simulink model "myexp5_3"  (R2022a)
settings: Solver=VariableStepAuto  StartTime=0.0  StopTime=100000  RelTol=1e-3
values from neighbouring files (symbols this model uses):
  M = n_list(i)    [exp5h.m]
libraries: commblkcod2 x2, commrandsrc3 x1, commchan3 x1, commsink2 x1
settings Model: Creator=惠普  LastModifiedBy=惠普

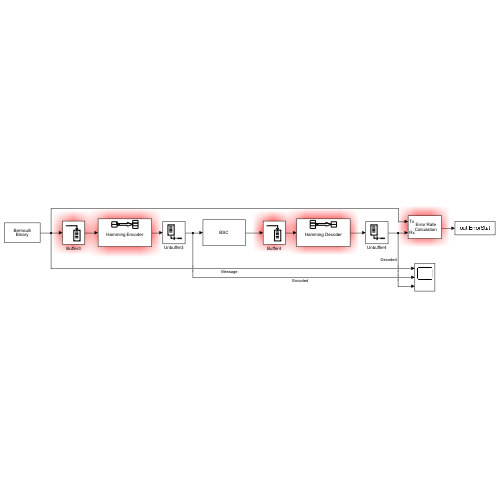
[thumbnail: Simulink's stored preview of the top-level diagram]
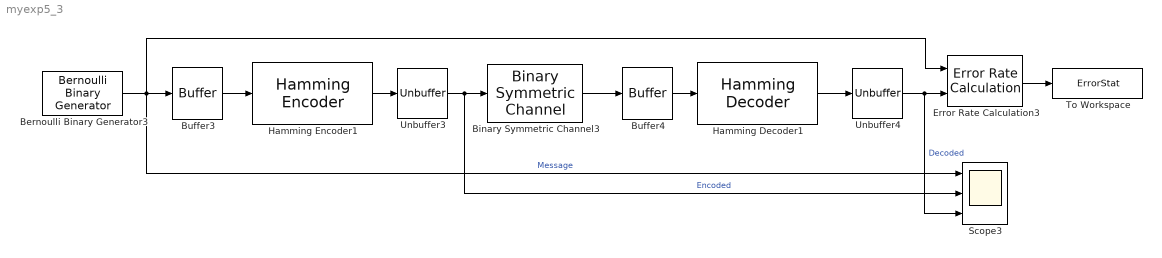
== system myexp5_3 ==
  Bernoulli Binary Generator3 : commrandsrc3/Bernoulli Binary Generator  ProbabilityOfZero=0.5  SeedSource=Auto  Seed=0  SampleTime=1  SamplesPerFrame=1  OutputDataType=double  SimulateUsing=Interpreted execution
  Binary Symmetric Channel3 : commchan3/Binary Symmetric Channel  ErrorProbability=eprob  ErrorVectorOutputPort=off  OutputDataType=double  OutputDataTypeSL=double  Seed=137  SimulateUsing=Code generation
      settings: SourceProductBaseCode=CM
  Buffer3 : Buffer  N=2^M-1-M  OutputFrames=off
  Buffer4 : Buffer  N=2^M-1  OutputFrames=off
  Error Rate Calculation3 : commsink2/Error Rate Calculation  N=2*(2^M-1-M)  st_delay=0  cp_mode=Entire frame  subframe=[]  PMode=Port  WsName=ErrorVec  RsMode2=off  stop=off  numErr=100  maxBits=1e6
  Hamming Decoder1 : commblkcod2/Hamming Decoder  n=2^M-1  k=2^M-1-M
      settings: SourceProductBaseCode=CM
  Hamming Encoder1 : commblkcod2/Hamming Encoder  n=2^M-1  k=2^M-1-M
      settings: SourceProductBaseCode=CM
  Scope3 : Scope  NumInputPorts=3
  To Workspace : ToWorkspace  VariableName=ErrorStat  SampleTime=-1
      settings: MaxDataPoints=1
  Unbuffer3 : Unbuffer
  Unbuffer4 : Unbuffer
  wires:
  Buffer4/1 -> Hamming Decoder1/1
  Buffer3/1 -> Hamming Encoder1/1
  Binary Symmetric Channel3/1 -> Buffer4/1
  Unbuffer4/1 -> Scope3/3, Error Rate Calculation3/2  "Decoded"
  Hamming Decoder1/1 -> Unbuffer4/1
  Unbuffer3/1 -> Scope3/2, Binary Symmetric Channel3/1  "Encoded"
  Bernoulli Binary Generator3/1 -> Scope3/1, Error Rate Calculation3/1, Buffer3/1  "Message"
  Hamming Encoder1/1 -> Unbuffer3/1
  Error Rate Calculation3/1 -> To Workspace/1
